simulink library "dsf"  (Simulink 8.1)
settings: Solver=ode45  StartTime=0.0  StopTime=10.0  RelTol=1e-3
settings Model: Creator=xsellart  LastModifiedBy=AT015555

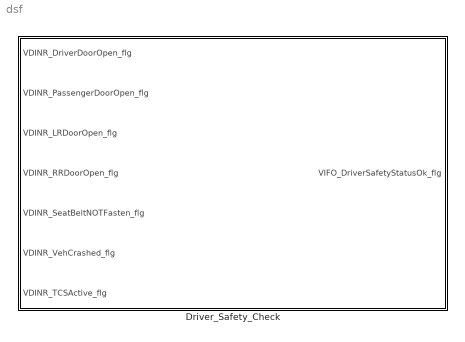
== system dsf ==
  Driver_Safety_Check : Subsystem

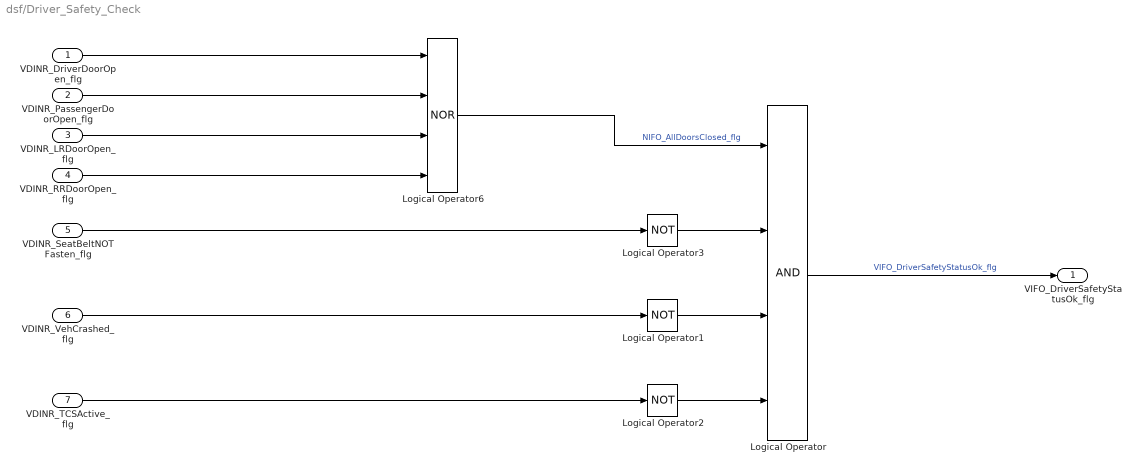
== system dsf/Driver_Safety_Check ==
  VDINR_DriverDoorOpen_flg : Inport
  VDINR_PassengerDoorOpen_flg : Inport  Port=2
  VDINR_LRDoorOpen_flg : Inport  Port=3
  VDINR_RRDoorOpen_flg : Inport  Port=4
  VDINR_SeatBeltNOTFasten_flg : Inport  Port=5
  VDINR_VehCrashed_flg : Inport  Port=6
  VDINR_TCSActive_flg : Inport  Port=7
  Logical Operator : Logic  Inputs=4  AllPortsSameDT=off  OutDataTypeStr=boolean
  Logical Operator1 : Logic  Operator=NOT  AllPortsSameDT=off  OutDataTypeStr=boolean
  Logical Operator2 : Logic  Operator=NOT  AllPortsSameDT=off  OutDataTypeStr=boolean
  Logical Operator3 : Logic  Operator=NOT  AllPortsSameDT=off  OutDataTypeStr=boolean
  Logical Operator6 : Logic  Operator=NOR  Inputs=4  AllPortsSameDT=off  OutDataTypeStr=boolean
  VIFO_DriverSafetyStatusOk_flg : Outport
  wires:
  VDINR_SeatBeltNOTFasten_flg/1 -> Logical Operator3/1
  Logical Operator/1 -> VIFO_DriverSafetyStatusOk_flg/1  "VIFO_DriverSafetyStatusOk_flg"
  VDINR_TCSActive_flg/1 -> Logical Operator2/1
  Logical Operator2/1 -> Logical Operator/4
  Logical Operator3/1 -> Logical Operator/2
  VDINR_VehCrashed_flg/1 -> Logical Operator1/1
  Logical Operator1/1 -> Logical Operator/3
  VDINR_RRDoorOpen_flg/1 -> Logical Operator6/4
  VDINR_LRDoorOpen_flg/1 -> Logical Operator6/3
  Logical Operator6/1 -> Logical Operator/1  "NIFO_AllDoorsClosed_flg"
  VDINR_PassengerDoorOpen_flg/1 -> Logical Operator6/2
  VDINR_DriverDoorOpen_flg/1 -> Logical Operator6/1
